simulink model "mSimpleConfigTest"  (R2019b)
settings: Solver=VariableStepAuto  StartTime=0.0  StopTime=10.0  RelTol=1e-3
undefined symbols (not defined in the file or in its folder): Var1
settings Model: DataDictionary=DdTestSimRunner.sldd  Creator=9bt  LastModifiedBy=4qz

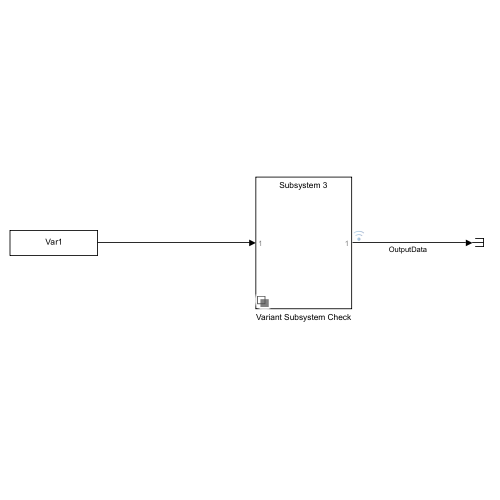
[thumbnail: Simulink's stored preview of the top-level diagram]
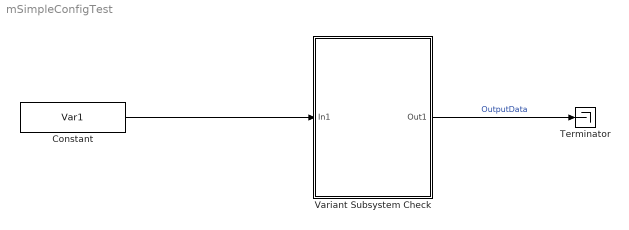
== system mSimpleConfigTest ==
  Constant : Constant  Value=Var1
  Terminator : Terminator
  Variant Subsystem Check : Subsystem  Variant=on  VariantControlMode=label  LabelModeActiveChoice=Choice_3
  wires:
  Constant/1 -> Variant Subsystem Check/1(In1)
  Variant Subsystem Check/1(Out1) -> Terminator/1  "OutputData"

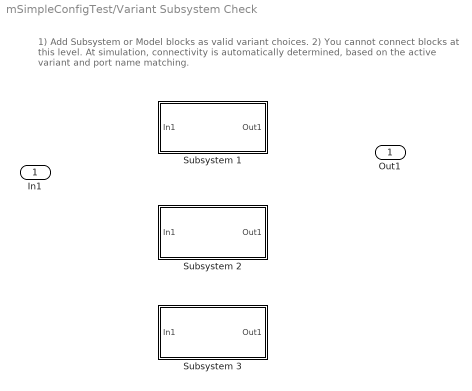
== system mSimpleConfigTest/Variant Subsystem Check ==
  note: 1) Add Subsystem or Model blocks as valid variant choices.
      | 2) You cannot connect blocks at this level. At simulation, connectivity is automatically
      | determined, based on the active variant and port name matching.
  In1 : Inport
  Subsystem 1 : Subsystem  VariantControl=Choice_1
  Subsystem 2 : Subsystem  VariantControl=Choice_2
  Subsystem 3 : Subsystem  VariantControl=Choice_3
  Out1 : Outport

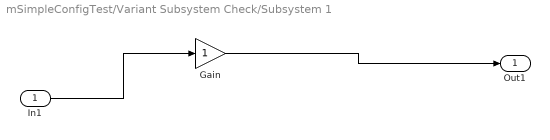
== system mSimpleConfigTest/Variant Subsystem Check/Subsystem 1 ==
  In1 : Inport
  Gain : Gain
  Out1 : Outport
  wires:
  Gain/1 -> Out1/1
  In1/1 -> Gain/1

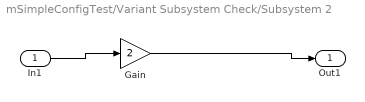
== system mSimpleConfigTest/Variant Subsystem Check/Subsystem 2 ==
  In1 : Inport
  Gain : Gain  Gain=2
  Out1 : Outport
  wires:
  In1/1 -> Gain/1
  Gain/1 -> Out1/1

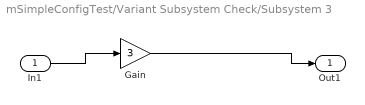
== system mSimpleConfigTest/Variant Subsystem Check/Subsystem 3 ==
  In1 : Inport
  Gain : Gain  Gain=3
  Out1 : Outport
  wires:
  In1/1 -> Gain/1
  Gain/1 -> Out1/1
